simulink model "motorPositionModel"  (R2021a)
settings: Solver=VariableStepAuto  StartTime=0.0  StopTime=10.0  RelTol=1e-3
undefined symbols (not defined in the file or in its folder): b, J, K, L, R
settings Model: Creator=Utkarsh Anand  LastModifiedBy=Utkarsh Anand
settings DataIOCC: SaveOutput=off  SaveTime=off

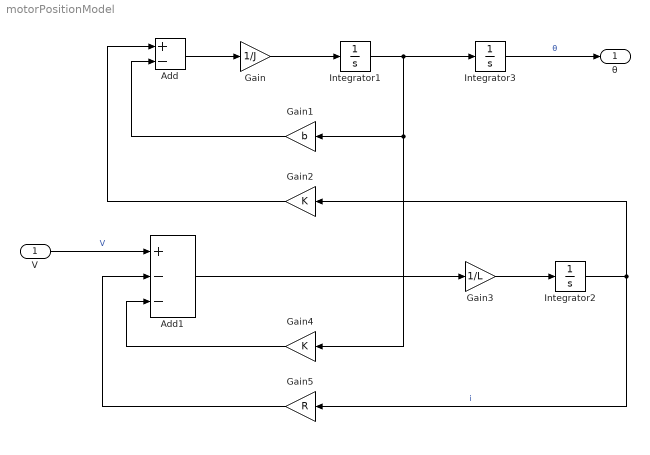
== system motorPositionModel ==
  V : Inport  OutDataTypeStr=double  PortDimensions=1  SampleTime=0
  Add : Sum  Inputs=+-
  Add1 : Sum  Inputs=+--
  Gain : Gain  Gain=1/J
  Gain1 : Gain  Gain=b
  Gain2 : Gain  Gain=K
  Gain3 : Gain  Gain=1/L
  Gain4 : Gain  Gain=K
  Gain5 : Gain  Gain=R
  Integrator1 : Integrator
  Integrator2 : Integrator
  Integrator3 : Integrator
  θ : Outport  OutDataTypeStr=double  PortDimensions=1  SampleTime=0
  wires:
  Gain/1 -> Integrator1/1
  Gain4/1 -> Add1/3
  Integrator2/1 -> Gain2/1, Gain5/1  "i"
  Add/1 -> Gain/1
  Gain5/1 -> Add1/2
  Add1/1 -> Gain3/1
  Gain1/1 -> Add/2
  Gain2/1 -> Add/1
  Integrator1/1 -> Gain1/1, Gain4/1, Integrator3/1
  Gain3/1 -> Integrator2/1
  V/1 -> Add1/1  "V"
  Integrator3/1 -> θ/1  "θ"
